simulink model "control"  (R2023a)
settings: Solver=VariableStepAuto  StartTime=0.0  StopTime=10.0  RelTol=1e-3
undefined symbols (not defined in the file): max_deg
libraries: fl_lib x3, nesl_utility x2, ee_lib x1
settings Model: Creator=tatyn  LastModifiedBy=tatyn

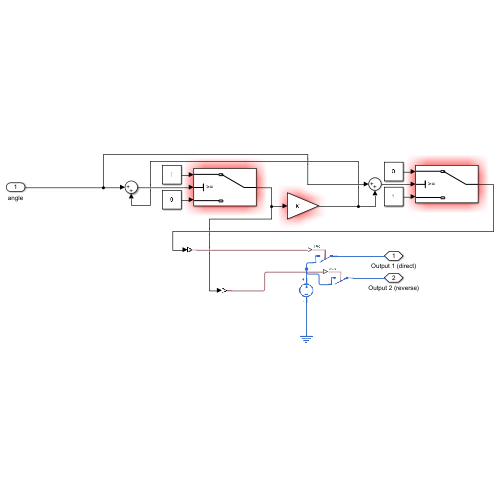
[thumbnail: Simulink's stored preview of the top-level diagram]
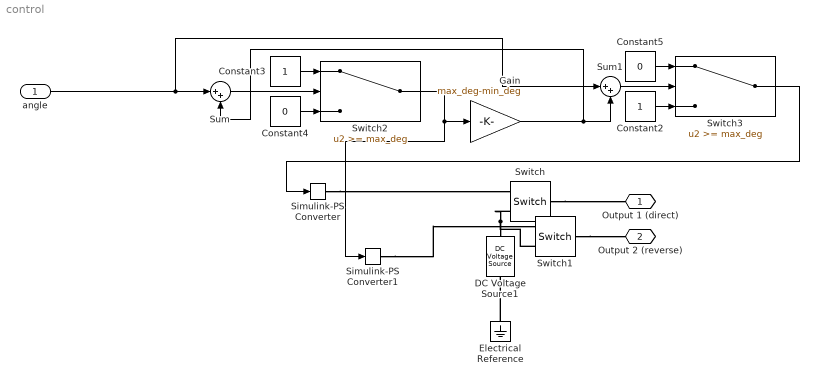
== system control ==
  angle : Inport
  Constant2 : Constant
  Constant3 : Constant
  Constant4 : Constant  Value=0
  Constant5 : Constant  Value=0
  DC Voltage Source1 : ee_lib/Additional Components/SPICE Sources/DC Voltage Source  DC=1 V
  Electrical Reference : fl_lib/Electrical/Electrical Elements/Electrical Reference
  Gain : Gain  Gain=max_deg-min_deg
  Simulink-PS Converter : nesl_utility/Simulink-PS Converter  PhysicalDomain=network_engine_domain  SubClassName=ps_input  LeftPortType=input  RightPortType=output  PseudoPeriodic=off  Frequencies=[]  NoiseDistribution=none  NoiseParameters=[]  Unit=1  AffineConversion=off  FilteringAndDerivatives=provide  SimscapeFilterOrder=1  InputFilterTimeConstant=0.001  UdotUserProvided=0
  Simulink-PS Converter1 : nesl_utility/Simulink-PS Converter  PhysicalDomain=network_engine_domain  SubClassName=ps_input  LeftPortType=input  RightPortType=output  PseudoPeriodic=off  Frequencies=[]  NoiseDistribution=none  NoiseParameters=[]  Unit=1  AffineConversion=off  FilteringAndDerivatives=provide  SimscapeFilterOrder=1  InputFilterTimeConstant=0.001  UdotUserProvided=0
  Sum : Sum  Inputs=|++
  Sum1 : Sum  Inputs=|++
  Switch : fl_lib/Electrical/Electrical Elements/Switch  R_closed=0.01 Ohm  G_open=1e-8 1/Ohm  Threshold=0.5  i_specify=off  i_priority=None  i=0 A  i_nominal_specify=off  i_nominal_unit=A  i_nominal_value=1  v_specify=off  v_priority=None  v=0 V  v_nominal_specify=off  v_nominal_unit=V  v_nominal_value=1
  Switch1 : fl_lib/Electrical/Electrical Elements/Switch  R_closed=0.01 Ohm  G_open=1e-8 1/Ohm  Threshold=0.5  i_specify=off  i_priority=None  i=0 A  i_nominal_specify=off  i_nominal_unit=A  i_nominal_value=1  v_specify=off  v_priority=None  v=0 V  v_nominal_specify=off  v_nominal_unit=V  v_nominal_value=1
  Switch2 : Switch  Threshold=max_deg  OutMin=0  OutMax=360  SaturateOnIntegerOverflow=off  InputSameDT=off
  Switch3 : Switch  Threshold=max_deg  OutMin=0  OutMax=360  SaturateOnIntegerOverflow=off  InputSameDT=off
  Output 1 (direct) : PMIOPort  Side=Right
  Output 2 (reverse) : PMIOPort  Port=2  Side=Right
  wires:
  Sum1/1 -> Switch3/2
  Sum/1 -> Switch2/2
  Constant5/1 -> Switch3/1
  Switch3/1 -> Simulink-PS Converter/1
  Gain/1 -> Sum1/2, Sum/2
  Switch2/1 -> Gain/1, Simulink-PS Converter1/1
  angle/1 -> Sum1/1, Sum/1
  Constant2/1 -> Switch3/3
  Constant4/1 -> Switch2/3
  Constant3/1 -> Switch2/1
  connections:
  DC Voltage Source1/LConn1 -- Switch/RConn2 -- Switch1/RConn2
  Switch1/LConn1 -- Output 2 (reverse)/RConn1
  Switch/LConn1 -- Output 1 (direct)/RConn1
  Simulink-PS Converter/RConn1 -- Switch/RConn1
  Simulink-PS Converter1/RConn1 -- Switch1/RConn1
  Electrical Reference/LConn1 -- DC Voltage Source1/RConn1
